simulink model "BLDC_Demo"  (R2019b)
settings: Solver=FixedStepDiscrete  StartTime=0.0  StopTime=Inf  FixedStep=0.001  RelTol=1e-3  EnableMultiTasking=on
PreLoadFcn:
  | run('BLDC_Demo_ini.m')
PostLoadFcn:
  | , if any(exist('dsrtsu_mdlpostloadfcn', 'file') ~= 0), dsrtsu_mdlpostloadfcn('Execute', bdroot); end,
InitFcn:
  | , if any(exist('rtifpga_mdlclblib', 'file') ~= 0), rtifpga_mdlclblib('Init', bdroot); end,
values from neighbouring files (symbols this model uses):
  BLDC_Ctrl_Ctrl_mode_SW = 3    [BLDC_Demo_ini.m]
  BLDC_Ctrl_iA_Set = 0    [BLDC_Demo_ini.m]
  BLDC_Ctrl_iA_Stroke = 0    [BLDC_Demo_ini.m]
  BLDC_Ctrl_is_dir = is_dir    [BLDC_Demo_ini.m]
  BLDC_Ctrl_is_index = is_index    [BLDC_Demo_ini.m]
  BLDC_Ctrl_Ki_iA = KI_i    (= 7190.04058695)    [BLDC_Demo_ini.m]
  BLDC_Ctrl_Ki_n = KI_n    (= 10.7018628664)    [BLDC_Demo_ini.m]
  BLDC_Ctrl_Kp_iA = KP_i    (= 3.09991410791)    [BLDC_Demo_ini.m]
  BLDC_Ctrl_Kp_n = KP_n    (= 0.0877769226706)    [BLDC_Demo_ini.m]
  BLDC_Ctrl_Limit_iA = IA_MAX    (= 9.5)    [BLDC_Demo_ini.m]
  BLDC_Ctrl_n_Limit = N_MAX    (= 3000)    [BLDC_Demo_ini.m]
  BLDC_Ctrl_n_Set = 0    [BLDC_Demo_ini.m]
  BLDC_Ctrl_n_Stroke = 0    [BLDC_Demo_ini.m]
  BLDC_Ctrl_TF_iA = TF_iA    (= 7.95774715459e-05)    [BLDC_Demo_ini.m]
  BLDC_Ctrl_TF_n = TF_n    (= 0.00159154943092)    [BLDC_Demo_ini.m]
  BLDC_Ctrl_v_Set = 0    [BLDC_Demo_ini.m]
  Modulator_Zi_HSD = Zi_HSD_LSD(:,4:6)    [BLDC_Demo_ini.m]
  Modulator_Zi_LSD = Zi_HSD_LSD(:,7:9)    [BLDC_Demo_ini.m]
  T_PWM = 50e-6    (= 5e-05)    [BLDC_Demo_ini.m]
undefined symbols (not defined in the file or in its folder): clock
libraries: simulink x29, rti1202lib_adc_class1 x8, dsextras x4, rtiemclib x4, rti1202lib_dio_class1 x3, rti1202lib_base x1
(part 2 of 3)

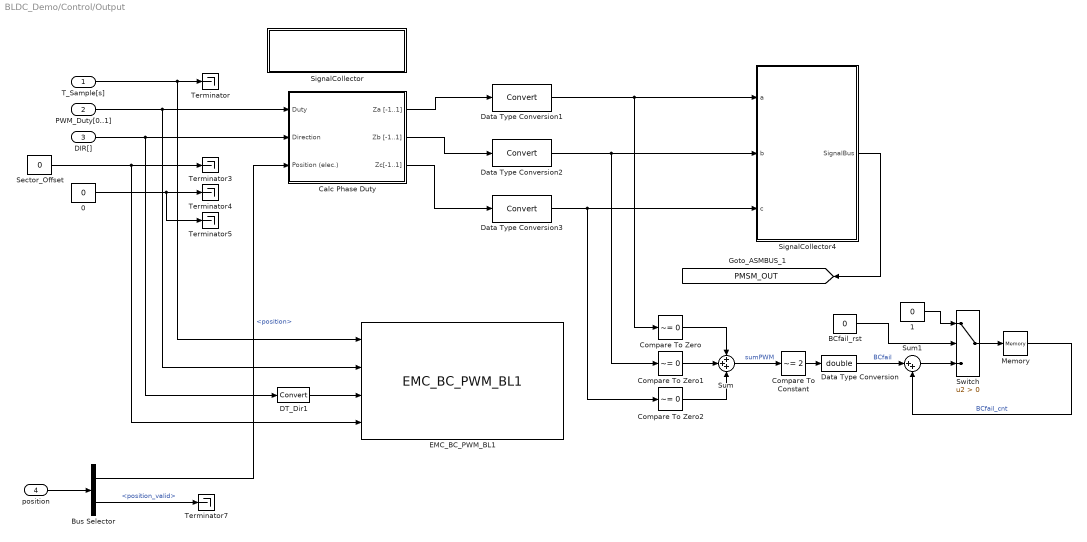
== system BLDC_Demo/Control/Output ==
  T_Sample[s] : Inport
  PWM_Duty[0..1] : Inport  Port=2
  DIR[] : Inport  Port=3
  position : Inport  Port=4
  0 : Constant  Value=0
  1 : Constant  Value=0
  BCfail_rst : Constant  Value=0
  Bus Selector : BusSelector  OutputSignals=position,position_valid
  Calc Phase Duty : Subsystem
  Compare To Constant : simulink/Logic and Bit Operations/Compare To Constant  relop=~=  const=2  OutDataTypeStr=uint8  ZeroCross=off
  Compare To Zero : simulink/Logic and Bit Operations/Compare To Zero  relop=~=  OutDataTypeStr=uint8  ZeroCross=off
  Compare To Zero1 : simulink/Logic and Bit Operations/Compare To Zero  relop=~=  OutDataTypeStr=uint8  ZeroCross=off
  Compare To Zero2 : simulink/Logic and Bit Operations/Compare To Zero  relop=~=  OutDataTypeStr=uint8  ZeroCross=off
  DT_Dir1 : DataTypeConversion
  Data Type Conversion : DataTypeConversion  OutDataTypeStr=double
  Data Type Conversion1 : DataTypeConversion
  Data Type Conversion2 : DataTypeConversion
  Data Type Conversion3 : DataTypeConversion
  EMC_BC_PWM_BL1 : rtiemclib/EMC_BC_PWM_BL1  DSProperties=struct('RTI',struct('Version',uint32(2),'BlockType',struct('isSLSource',uint8(0),'isSLSink',uint8(1),'isHWSource',uint8(0),'isHWSink',uint8(1),'isSetup',uint8(0),'isInline',uint8(1),'isNonInline',uint8(0),'isInterrupt',uint8(0),'isChannelwise',uint8(0)),'IOBoardType','DSEMC','UnitType','BCPWM','Identifier','BCPWM','DialogType','ML','BlockSet','RTIEMC','SlaveProcessor','NONE'))  RTIBlockInterface=struct('InputPortsWidth',int32([1 1 1 1 1 1 1 1]),'InputPortsActive',[1 1 1 1 0 0 0 0],'InputPortsName',{{'Period',['Duty Cycle'],'Direction','Offset','Position',['Position Valid'],['Specific Pattern'],['Output Enable']}},'InputPortsDataType',{{'SS_DOUBLE','SS_DOUBLE','SS_INT32','SS_DOUBLE','SS_DOUBLE','SS_BOOLEAN','SS_UINT32','SS_BOOLEAN'}},'BlockDisplay',{{['EMC Block Commutated PWM\nUnit: 1\nPort: 1\nChannel: 7'],'center'}},'IconTransparency','on','InitLevel',3,'DialogFcn','rtiemcbcpwmgui','BlockName',struct('Token',{{'EMC_BC_PWM_BL1'}}))  RTIBlockParameters=struct('UnitNo',{{1,'OFF',[1 2]}},'PortNo',{{1,'OFF',[1 3]}},'ChannelNo',{{7,'OFF',[1 14]}},'HighLevel',{{3,'OFF',[1 3]}},'PhaseAPos',{{[3 3 1 1 1 1],'OFF',[1 6]}},'PhaseANeg',{{[1 1 1 3 3 1],'OFF',[1 6]}},'PhaseBPos',{{[1 1 3 3 1 1],'OFF',[1 6]}},'PhaseBNeg',{{[3 1 1 1 1 3],'OFF',[1 6]}},'PhaseCPos',{{[1 1 1 1 3 3],'OFF',[1 6]}},'PhaseCNeg',{{[1 3 3 1 1 1],'OFF',[1 6]}},'UpdateMode',{{1,'OFF',[1 3]}},'DeadTime',{{'0','OFF',[0 0.000655]}},'InitPeriod',{{'5e-05','OFF',[1e-7 1.34]}},'InitDutyCycle',{{'0.5','OFF',[0 1]}},'PhaseAPosInit',{{1,'OFF',[1 2]}},'PhaseANegInit',{{1,'OFF',[1 2]}},'PhaseBPosInit',{{1,'OFF',[1 2]}},'PhaseBNegInit',{{1,'OFF',[1 2]}},'PhaseCPosInit',{{1,'OFF',[1 2]}},'PhaseCNegInit',{{1,'OFF',[1 2]}},'TerminationMode',{{0,'OFF',[0 1]}},'PhaseAPosTerm',{{1,'OFF',[1 2]}},'PhaseANegTerm',{{1,'OFF',[1 2]}},'PhaseBPosTerm',{{1,'OFF',[1 2]}},'PhaseBNegTerm',{{1,'OFF',[1 2]}},'PhaseCPosTerm',{{1,'OFF',[1 2]}},'PhaseCNegTerm',{{1,'OFF',[1 2]}},'SectorOffset',{{'0','OFF',[-60 60]}},'EnableSectorOffsetPort',{{1,'OFF',[0 1]}},'EnablePositionPort',{{1,'OFF',[1 2]}},'EnableDirectionPort',{{1,'OFF',[0 1]}},'InitDirection',{{1,'OFF',[-1 1]}},'AcuInstanceIdx',{{1,'OFF',[1 4]}},'EnableEvent',{{1,'OFF',[0 1]}},'EventMode',{{3,'OFF',[1 3]}},'EventOnStart',{{0,'OFF',[0 1]}},'EventOnCenter',{{1,'OFF',[0 1]}},'EventDelay',{{'0','OFF',[0 1.34]}},'EventRate',{{'1','OFF',[1 256]}},'TriggerLine',{{1,'OFF',[1 16]}},'TLCFileName',{{'rtiemcbcpwm','OFF',[]}},'ValidateEventBuildCheck',{{true,'OFF',[]}},'EnableSpecificPatternPort',{{0,'OFF',[0 1]}},'PhaseAPosSpecPatt',{{[1 1 1 1 1 1],'OFF',[1 6]}},'PhaseANegSpecPatt',{{[1 1 1 1 1 1],'OFF',[1 6]}},'PhaseBPosSpecPatt',{{[1 1 1 1 1 1],'OFF',[1 6]}},'PhaseBNegSpecPatt',{{[1 1 1 1 1 1],'OFF',[1 6]}},'PhaseCPosSpecPatt',{{[1 1 1 1 1 1],'OFF',[1 6]}},'PhaseCNegSpecPatt',{{[1 1 1 1 1 1],'OFF',[1 6]}},'ActivateOutputEnablePort',{{0,'OFF',[0 1]}},'InitOutputEnable',{{1,'OFF',[1 2]}})  RTISFcnParameters=struct('UnitNo','int32','PortNo','int32','ChannelNo','int32','HighLevel','int32','PhaseAPos','int32','PhaseANeg','int32','PhaseBPos','int32','PhaseBNeg','int32','PhaseCPos','int32','PhaseCNeg','int32','UpdateMode','int32','DeadTime','double','InitPeriod','double','InitDutyCycle','double','PhaseAPosInit','int32','PhaseANegInit','int32','PhaseBPosInit','int32','PhaseBNegInit','int32','PhaseCPosInit','int32','PhaseCNegInit','int32','TerminationMode','int32','PhaseAPosTerm','int32','PhaseANegTerm','int32','PhaseBPosTerm','int32','PhaseBNegTerm','int32','PhaseCPosTerm','int32','PhaseCNegTerm','int32','SectorOffset','double','EnableSectorOffsetPort','int32','EnablePositionPort','int32','EnableDirectionPort','int32','InitDirection','int32','AcuInstanceIdx','int32','EnableEvent','int32','EventMode','int32','EventOnStart','int32','EventOnCenter','int32','EventDelay','double','EventRate','int32','TriggerLine','int32','TLCFileName','char','EnableSpecificPatternPort','int32','PhaseAPosSpecPatt','int32','PhaseANegSpecPatt','int32','PhaseBPosSpecPatt','int32','PhaseBNegSpecPatt','int32','PhaseCPosSpecPatt','int32','PhaseCNegSpecPatt','int32','ActivateOutputEnablePort','int32','InitOutputEnable','int32')  RTIBlockParaDefault=struct('UnitNo',1,'PortNo',1,'ChannelNo',1,'HighLevel',1,'PhaseAPos',[3 3 1 1 1 1],'PhaseANeg',[1 1 1 3 3 1],'PhaseBPos',[1 1 3 3 1 1],'PhaseBNeg',[3 1 1 1 1 3],'PhaseCPos',[1 1 1 1 3 3],'PhaseCNeg',[1 3 3 1 1 1],'UpdateMode',1,'DeadTime',0,'InitPeriod',5e-5,'InitDutyCycle',2^-1,'PhaseAPosInit',1,'PhaseANegInit',1,'PhaseBPosInit',1,'PhaseBNegInit',1,'PhaseCPosInit',1,'PhaseCNegInit',1,'TerminationMode',0,'PhaseAPosTerm',1,'PhaseANegTerm',1,'PhaseBPosTerm',1,'PhaseBNegTerm',1,'PhaseCPosTerm',1,'PhaseCNegTerm',1,'SectorOffset',0,'EnableSectorOffsetPort',0,'EnablePositionPort',1,'EnableDirectionPort',0,'InitDirection',1,'AcuInstanceIdx',0,'EnableEvent',0,'EventMode',1,'EventOnStart',1,'EventOnCenter',0,'EventDelay',0,'EventRate',1,'TriggerLine',1,'TLCFileName','rtiemcbcpwm','ValidateEventBuildCheck',0,'EnableSpecificPatternPort',0,'PhaseAPosSpecPatt',[1 1 1 1 1 1],'PhaseANegSpecPatt',[1 1 1 1 1 1],'PhaseBPosSpecPatt',[1 1 1 1 1 1],'PhaseBNegSpecPatt',[1 1 1 1 1 1],'PhaseCPosSpecPatt',[1 1 1 1 1 1],'PhaseCNegSpecPatt',[1 1 1 1 1 1],'ActivateOutputEnablePort',0,'InitOutputEnable',1)
      settings: SourceProductName=dSPACE RTI Electric Motor Control Blockset
  Memory : Memory  InheritSampleTime=on
  Sector_Offset : Constant  Value=0
  SignalCollector : Subsystem
  SignalCollector4 : Subsystem
  Sum : Sum  Inputs=+++
  Sum1 : Sum  Inputs=|++
  Switch : Switch  Criteria=u2 > Threshold
  Terminator{,3..5,7} (5 alike) : Terminator
  tag scope: PMSM_OUT=global
  wires:
  PWM_Duty[0..1]/1 -> EMC_BC_PWM_BL1/2, Calc Phase Duty/1(Duty)
  T_Sample[s]/1 -> EMC_BC_PWM_BL1/1, Terminator/1
  SignalCollector4/1(SignalBus) -> [PMSM_OUT]
  DIR[]/1 -> DT_Dir1/1, Calc Phase Duty/2(Direction)
  Sector_Offset/1 -> Terminator3/1, EMC_BC_PWM_BL1/4
  0/1 -> Terminator5/1, Terminator4/1
  Compare To Zero1/1 -> Sum/2
  Compare To Zero/1 -> Sum/1
  Compare To Zero2/1 -> Sum/3
  Sum/1 -> Compare To Constant/1  "sumPWM"
  Compare To Constant/1 -> Data Type Conversion/1
  Memory/1 -> Sum1/2  "BCfail_cnt"
  Data Type Conversion/1 -> Sum1/1  "BCfail"
  Sum1/1 -> Switch/3
  Switch/1 -> Memory/1
  1/1 -> Switch/1
  BCfail_rst/1 -> Switch/2
  Data Type Conversion1/1 -> SignalCollector4/1(a), Compare To Zero/1
  Data Type Conversion2/1 -> SignalCollector4/2(b), Compare To Zero1/1
  Data Type Conversion3/1 -> SignalCollector4/3(c), Compare To Zero2/1
  DT_Dir1/1 -> EMC_BC_PWM_BL1/3
  position/1 -> Bus Selector/1
  Bus Selector/2 -> Terminator7/1  "<position_valid>"
  Bus Selector/1 -> Calc Phase Duty/3(Position (elec.))  "<position>"
  Calc Phase Duty/1(Za [-1..1]) -> Data Type Conversion1/1
  Calc Phase Duty/2(Zb [-1..1]) -> Data Type Conversion2/1
  Calc Phase Duty/3(Zc[-1..1]) -> Data Type Conversion3/1

== system BLDC_Demo/Control/bldc_ctrl_par_sig ==
  rect_pulse : Inport
  MDL_DISP : Subsystem
      mask Display: disp('Simulation results:\nArbitrary input to\nControlDesk from MDL')
  MDL_DISP_INPUT : Subsystem
      mask Display: disp('Simulation results:\nArbitrary input to\nControlDesk from MDL')
  MDL_OUTPUT : Subsystem
      mask Display: disp('Simulation results:\nArbitrary input to\nControlDesk from MDL')
  MDL_PAR : Subsystem
      mask Display: disp('Simulation parameters:\nContinuous output from\nControlDesk to MDL')
  wires:
  rect_pulse/1 -> MDL_PAR/1(rect_pulse)

== system BLDC_Demo/RTI Data/RTI Data Store ==
  RTI Data Store : Subsystem  mask(RTI_DATA_STORE){}
      mask help:
      | RTI Data Store Block. This block is used by RTI to store internal model dependent data. Deleting this block will result in data loss.
      |
      | NEVER DELETE, COPY, OR MODIFY THIS BLOCK!
      mask Help:
      | RTI Data Store Block. This block is used by RTI to store internal model dependent data. Deleting this block will result in data loss.
      | 
      | NEVER DELETE, COPY, OR MODIFY THIS BLOCK!
      mask Display: text(0.5, 0.5, ' ', 'HorizontalAlignment', 'center');

== system BLDC_Demo/Ref_value_gen/Enabled and Triggered Subsystem ==
  n_ref : Inport
  Constant : Constant
  Constant1 : Constant  Value=0
  Hit Crossing : HitCross  HitCrossingOffset=0.5  HitCrossingDirection=rising
  Memory : Memory  InheritSampleTime=on
  Product : Product  RndMeth=Zero
  Relational Operator : RelationalOperator  Operator=<=  OutDataTypeStr=boolean  RndMeth=Nearest
  Relational Operator1 : RelationalOperator  OutDataTypeStr=boolean  RndMeth=Nearest
  Sum : Sum  Inputs=|++
  Switch : Switch  Threshold=0.5
  Switch1 : Switch  Threshold=0.5
  load_signal_0 : Constant  Value=0
  load_signal_generator : Constant
  start_time_samples : Constant  Value=1000
  switch_out_boarder : Constant  Value=0.5
  load_ref : Outport  VectorParamsAs1DForOutWhenUnconnected=off
  wires:
  Constant/1 -> Sum/1
  Sum/1 -> Switch/3
  Constant1/1 -> Switch/1
  Switch/1 -> Relational Operator/1, Memory/1
  Hit Crossing/1 -> Switch/2
  n_ref/1 -> Hit Crossing/1, Relational Operator1/1
  start_time_samples/1 -> Relational Operator/2
  load_signal_0/1 -> Switch1/1
  Relational Operator/1 -> Switch1/2
  load_signal_generator/1 -> Switch1/3
  Switch1/1 -> Product/2
  switch_out_boarder/1 -> Relational Operator1/2
  Product/1 -> load_ref/1
  Relational Operator1/1 -> Product/1
  Memory/1 -> Sum/2

== system BLDC_Demo/Control/Control_load_machine/duty_cycle_2_torque ==
  In_duty_cycle[0..1] : Inport
  Divide : Product  Inputs=*/
  coil_resistance : Constant  Value=24
  current_2_load1 : Lookup_n-D  NumberOfTableDimensions=1  BreakpointsForDimension1=[0, 0.05, 0.1, 0.2, 0.3, 0.4]  Table=[0, 0.05, 0.2, 0.7, 1.4, 1.9]  InputSameDT=on
  duty_cycle_2_voltage : Subsystem
  Out_torque[Nm] : Outport  VectorParamsAs1DForOutWhenUnconnected=off
  wires:
  In_duty_cycle[0..1]/1 -> duty_cycle_2_voltage/1(In_duty_cycle[0..1])
  duty_cycle_2_voltage/1(Out_duty_voltage[V]) -> Divide/1
  coil_resistance/1 -> Divide/2
  current_2_load1/1 -> Out_torque[Nm]/1
  Divide/1 -> current_2_load1/1

== system BLDC_Demo/Control/Control_load_machine/torque_2_duty_cycle ==
  In_torque[Nm] : Inport
  current_2_voltage : Gain  Gain=24
  load_2_current4 : Lookup_n-D  NumberOfTableDimensions=1  BreakpointsForDimension1=[0, 0.05, 0.2, 0.7, 1.4, 1.9]  Table=[0, 0.05, 0.1, 0.2, 0.3, 0.4]  InputSameDT=on
  voltage_2_duty_cycle : Subsystem
  Out_duty_cycle[0..1] : Outport  VectorParamsAs1DForOutWhenUnconnected=off
  wires:
  load_2_current4/1 -> current_2_voltage/1
  current_2_voltage/1 -> voltage_2_duty_cycle/1(In_voltage[V])
  In_torque[Nm]/1 -> load_2_current4/1
  voltage_2_duty_cycle/1(Out_duty_cycle) -> Out_duty_cycle[0..1]/1

== system BLDC_Demo/Control/Control_load_machine/torque_2_duty_cycle1 ==
  In_torque[Nm] : Inport
  current_2_voltage : Gain  Gain=24
  load_2_current4 : Lookup_n-D  NumberOfTableDimensions=1  BreakpointsForDimension1=[0, 0.05, 0.2, 0.7, 1.4, 1.9]  Table=[0, 0.05, 0.1, 0.2, 0.3, 0.4]  InputSameDT=on
  voltage_2_duty_cycle : Subsystem
  Out_duty_cycle[0..1] : Outport  VectorParamsAs1DForOutWhenUnconnected=off
  wires:
  voltage_2_duty_cycle/1(Out_duty_cycle[0..1]) -> Out_duty_cycle[0..1]/1
  In_torque[Nm]/1 -> load_2_current4/1
  current_2_voltage/1 -> voltage_2_duty_cycle/1(In_voltage[V])
  load_2_current4/1 -> current_2_voltage/1

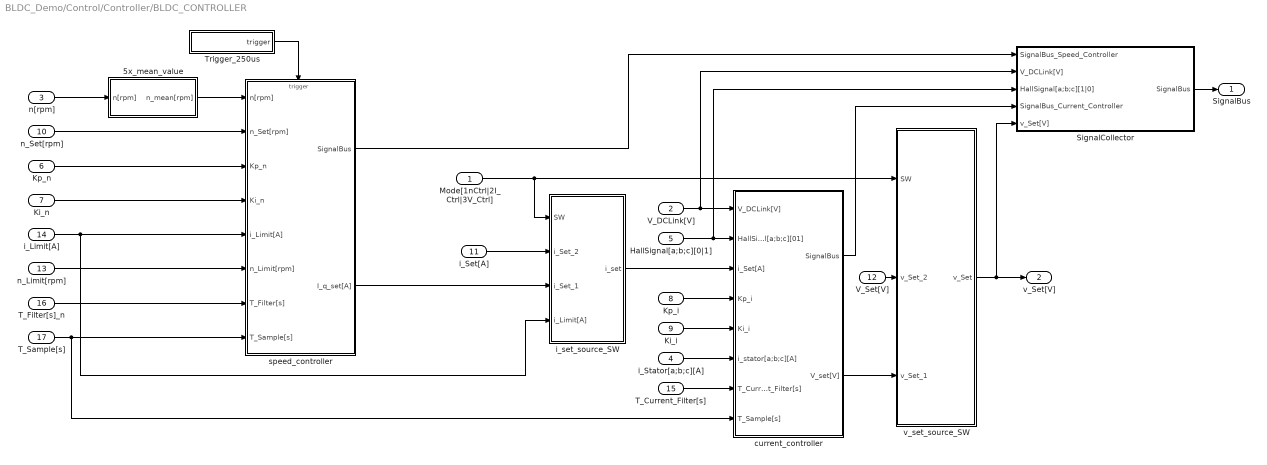
== system BLDC_Demo/Control/Controller/BLDC_CONTROLLER ==
  Mode[1nCtrl|2I_Ctrl|3V_Ctrl] : Inport
  V_DCLink[V] : Inport  Port=2
  n[rpm] : Inport  Port=3
  i_Stator[a;b;c][A] : Inport  Port=4
  HallSignal[a;b;c][0|1] : Inport  Port=5
  Kp_n : Inport  Port=6
  Ki_n : Inport  Port=7
  Kp_i : Inport  Port=8
  Ki_i : Inport  Port=9
  n_Set[rpm] : Inport  Port=10
  i_Set[A] : Inport  Port=11
  V_Set[V] : Inport  Port=12
  n_Limit[rpm] : Inport  Port=13
  i_Limit[A] : Inport  Port=14
  T_Current_Filter[s] : Inport  Port=15
  T_Filter[s]_n : Inport  Port=16
  T_Sample[s] : Inport  Port=17
  5x_mean_value : Subsystem
  SignalCollector : Subsystem
  Trigger_250us : Subsystem
  current_controller : Subsystem
  i_set_source_SW : Subsystem
  speed_controller : Subsystem
  v_set_source_SW : Subsystem
  SignalBus : Outport  VectorParamsAs1DForOutWhenUnconnected=off
  v_Set[V] : Outport  Port=2  VectorParamsAs1DForOutWhenUnconnected=off
  wires:
  T_Sample[s]/1 -> current_controller/8(T_Sample[s]), speed_controller/8(T_Sample[s])
  i_Limit[A]/1 -> i_set_source_SW/4(i_Limit[A]), speed_controller/5(i_Limit[A])
  Ki_n/1 -> speed_controller/4(Ki_n)
  Kp_n/1 -> speed_controller/3(Kp_n)
  n[rpm]/1 -> 5x_mean_value/1(n[rpm])
  n_Set[rpm]/1 -> speed_controller/2(n_Set[rpm])
  n_Limit[rpm]/1 -> speed_controller/6(n_Limit[rpm])
  V_DCLink[V]/1 -> SignalCollector/2(V_DCLink[V]), current_controller/1(V_DCLink[V])
  T_Current_Filter[s]/1 -> current_controller/7(T_Current_Filter[s])
  HallSignal[a;b;c][0|1]/1 -> SignalCollector/3(HallSignal[a;b;c][1|0]), current_controller/2(HallSignal[a;b;c][01])
  i_Stator[a;b;c][A]/1 -> current_controller/6(i_stator[a;b;c][A])
  v_set_source_SW/1(v_Set) -> v_Set[V]/1, SignalCollector/5(v_Set[V])
  current_controller/2(" V_set[V]") -> v_set_source_SW/3(v_Set_1)
  V_Set[V]/1 -> v_set_source_SW/2(v_Set_2)
  speed_controller/2(I_q_set[A]) -> i_set_source_SW/3(i_Set_1)
  i_Set[A]/1 -> i_set_source_SW/2(i_Set_2)
  Ki_i/1 -> current_controller/5(Ki_i)
  Kp_i/1 -> current_controller/4(Kp_i)
  SignalCollector/1(SignalBus) -> SignalBus/1
  i_set_source_SW/1(i_set) -> current_controller/3(i_Set[A])
  Mode[1nCtrl|2I_Ctrl|3V_Ctrl]/1 -> i_set_source_SW/1(SW), v_set_source_SW/1(SW)
  current_controller/1(SignalBus) -> SignalCollector/4(SignalBus_Current_Controller)
  speed_controller/1(SignalBus) -> SignalCollector/1(SignalBus_Speed_Controller)
  T_Filter[s]_n/1 -> speed_controller/7(T_Filter[s])
  5x_mean_value/1(n_mean[rpm]) -> speed_controller/1(n[rpm])
  Trigger_250us/1(trigger) -> speed_controller/Trigger

== system BLDC_Demo/Control/Controller/BLOCK_MODULATOR ==
  V_DCLink[V] : Inport
  v_Set[V] : Inport  Port=2
  HallSignal[a;b;c][0|1] : Inport  Port=3
  Data Type Conversion : DataTypeConversion  OutDataTypeStr=double
  Data Type Conversion1 : DataTypeConversion  OutDataTypeStr=double
  DutyCycle : Subsystem
  Label_DutyCycle_HSD[a;b;c][0_1] : Subsystem
  Label_DutyCycle_LSD[a;b;c][0_1] : Subsystem
  Product1 : Product  RndMeth=Zero
  SignalCollector : Subsystem
  SwitchHSD : Switch
  SwitchLSD : Switch
  Zabc_HSD : CombinatorialLogic  TruthTable=Zi_HSD
  Zabc_LSD : CombinatorialLogic  TruthTable=Zi_LSD
  SignalBus : Outport  VectorParamsAs1DForOutWhenUnconnected=off
  d[0_1] : Outport  Port=2  VectorParamsAs1DForOutWhenUnconnected=off
  DIR : Outport  Port=3  VectorParamsAs1DForOutWhenUnconnected=off
  wires:
  v_Set[V]/1 -> DutyCycle/1(v_set[V])
  V_DCLink[V]/1 -> DutyCycle/2(V_DCLink[V])
  DutyCycle/2(DIR) -> SwitchHSD/2, SwitchLSD/2, SignalCollector/2(DIR), DIR/1
  DutyCycle/1(d[0_1]) -> Product1/1, SignalCollector/1(d[0_1]), d[0_1]/1
  SignalCollector/1(SignalBus) -> SignalBus/1
  HallSignal[a;b;c][0|1]/1 -> Zabc_HSD/1, Zabc_LSD/1
  Zabc_LSD/1 -> Data Type Conversion/1
  Zabc_HSD/1 -> Data Type Conversion1/1
  SwitchHSD/1 -> Product1/2
  Data Type Conversion/1 -> SwitchLSD/1, SwitchHSD/3
  Data Type Conversion1/1 -> SwitchHSD/1, SwitchLSD/3
  Label_DutyCycle_HSD[a;b;c][0_1]/1(Out) -> SignalCollector/3(DutyCycle_HSD[a;b;c][0_1])
  Label_DutyCycle_LSD[a;b;c][0_1]/1(Out) -> SignalCollector/4(DutyCycle_LSD[a;b;c][0_1])
  Product1/1 -> Label_DutyCycle_HSD[a;b;c][0_1]/1(In)
  SwitchLSD/1 -> Label_DutyCycle_LSD[a;b;c][0_1]/1(In)

== system BLDC_Demo/Control/Controller/SignalCollector ==
  BusCreator : BusCreator  Inputs=1
  tag scope: Controller_Bus=global
  wires:
  [PMSM_CONTROLLER] -> BusCreator/1
  BusCreator/1 -> [Controller_Bus]  "Controller"

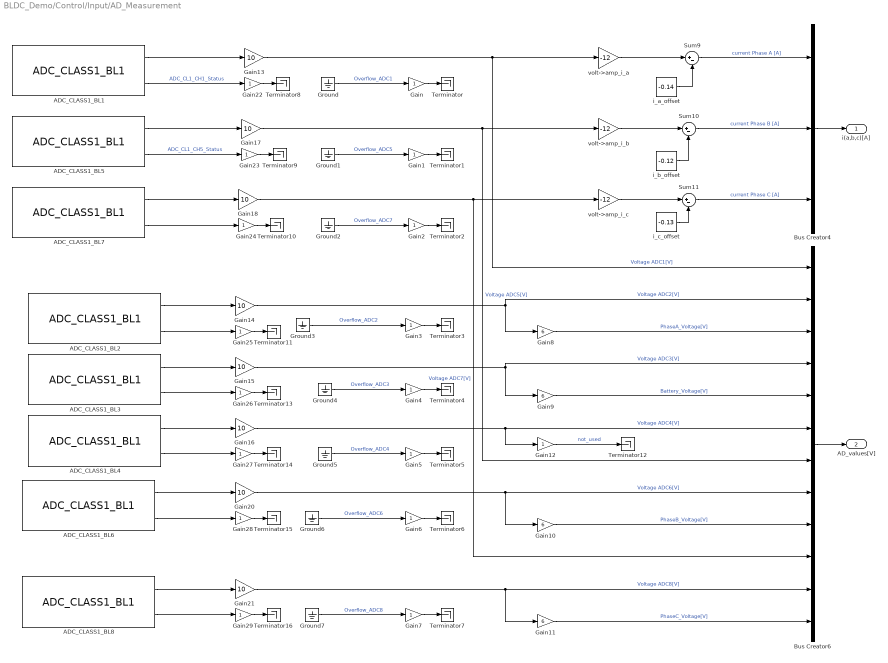
== system BLDC_Demo/Control/Input/AD_Measurement ==
  " i_a_offset" : Constant  Value=-0.14
  " i_b_offset  " : Constant  Value=-0.12
  ADC_CLASS1_BL1 : rti1202lib_adc_class1/ADC_CLASS1_BL1  DSProperties=struct('RTI',struct('Version',uint32(1),'BlockType',struct('isSLSource',uint8(1),'isSLSink',uint8(1),'isHWSource',uint8(0),'isHWSink',uint8(1),'isSetup',uint8(0),'isInline',uint8(1),'isNonInline',uint8(0),'isInterrupt',uint8(0),'isChannelwise',uint8(1)),'IOBoardType',{{'DS120X','STD','ADCC1'}},'UnitType','ADC','Identifier','ADC','DialogType','ML','BlockSet','NONE','SlaveProcessor','NONE'))  RTIBlockInterface=struct('InputPortsActive',0,'InputPortsWidth',int32(1),'InputPortsDataType',{{'SS_BOOLEAN'}},'InputPortsName',{{'Continue'}},'OutputPortsActive',[1 1],'OutputPortsWidth',int32([1 1]),'OutputPortsDataType',{{'SS_DOUBLE','SS_INT16'}},'OutputPortsName',{{'ADC','Status'}},'DialogFcn','rti120xstdadcc1adcgui','SampleTime',{{-1}},'InitLevel',3,'IconTransparency','on','BlockDisplay',{{['ADC CL1\nChannel: 1'],'center'}},'BlockName',struct('Token',{{'ADC_CLASS1_BL1'}}))  RTIBlockParameters=struct('ReadMode',{{2,'OFF',[1 2]}},'ChannelNo',{{1,'OFF',[]}},'ConversionMode',{{1,'OFF',[1 2]}},'TriggerSource',{{2,'OFF',[1 2]}},'TriggerLineIn',{{1,'OFF',[1 16]}},'SampleMode',{{1,'OFF',[1 2]}},'BurstTriggerSource',{{1,'OFF',[1 2]}},'BurstTriggerLine',{{1,'OFF',[1 16]}},'ConvTriggerSource',{{3,'OFF',[1 3]}},'ConvTriggerLine',{{1,'OFF',[1 16]}},'ConvPeriod',{{'100e-6','OFF',[1e-6 1.34]}},'ConvPeriodCheck',{{0,'OFF',[]}},'BurstSize',{{'10','OFF',[]}},'BurstSizeCheck',{{0,'OFF',[]}},'DataSetOffset',{{'0','OFF',[]}},'DataSetOffsetCheck',{{0,'OFF',[]}},'DataSetLength',{{'1','OFF',[]}},'DataSetLengthCheck',{{0,'OFF',[]}},'EnableTriggerEvent',{{0,'OFF',[0 1]}},'TriggerMode',{{2,'OFF',[1 3]}},'TriggerLineOut',{{1,'OFF',[1 16]}},'ADCSWStartEnable',{{0,'OFF',[0 1]}},'SampleTime',{{'-1','OFF',[-1 inf]}},'SampleTimeCheck',{{0,'OFF',[]}},'StatusPortEnable',{{1,'OFF',[0 1]}},'TLCFileName',{{'rti120xadc_c1_adc','OFF',[]}})  RTISFcnParameters=struct('ReadMode','int16','ChannelNo','int16','ConversionMode','int16','TriggerSource','int16','TriggerLineIn','int16','SampleMode','int16','BurstTriggerSource','int16','BurstTriggerLine','int16','ConvTriggerSource','int16','ConvTriggerLine','int16','ConvPeriod','double','BurstSize','int16','DataSetOffset','int16','DataSetLength','int16','EnableTriggerEvent','int16','TriggerMode','int16','TriggerLineOut','int16','ADCSWStartEnable','int16','SampleTime','double','StatusPortEnable','int16','TLCFileName','char')  RTIBlockParaDefault=struct('ReadMode',1,'ChannelNo',1,'ConversionMode',1,'TriggerSource',1,'TriggerLineIn',1,'SampleMode',1,'BurstTriggerSource',1,'BurstTriggerLine',1,'ConvTriggerSource',3,'ConvTriggerLine',1,'ConvPeriod',0.0001,'ConvPeriodCheck',0,'BurstSize',10,'BurstSizeCheck',0,'DataSetOffset',0,'DataSetOffsetCheck',0,'DataSetLength',1,'DataSetLengthCheck',0,'EnableTriggerEvent',0,'TriggerMode',2,'TriggerLineOut',1,'ADCSWStartEnable',0,'SampleTime',-1,'SampleTimeCheck',1,'StatusPortEnable',0,'TLCFileName','rti120xadc_c1_adc')
  ADC_CLASS1_BL2 : rti1202lib_adc_class1/ADC_CLASS1_BL1  DSProperties=struct('RTI',struct('Version',uint32(1),'BlockType',struct('isSLSource',uint8(1),'isSLSink',uint8(1),'isHWSource',uint8(0),'isHWSink',uint8(1),'isSetup',uint8(0),'isInline',uint8(1),'isNonInline',uint8(0),'isInterrupt',uint8(0),'isChannelwise',uint8(1)),'IOBoardType',{{'DS120X','STD','ADCC1'}},'UnitType','ADC','Identifier','ADC','DialogType','ML','BlockSet','NONE','SlaveProcessor','NONE'))  RTIBlockInterface=struct('InputPortsActive',0,'InputPortsWidth',int32(1),'InputPortsDataType',{{'SS_BOOLEAN'}},'InputPortsName',{{'Continue'}},'OutputPortsActive',[1 1],'OutputPortsWidth',int32([1 1]),'OutputPortsDataType',{{'SS_DOUBLE','SS_INT16'}},'OutputPortsName',{{'ADC','Status'}},'DialogFcn','rti120xstdadcc1adcgui','SampleTime',{{-1}},'InitLevel',3,'IconTransparency','on','BlockDisplay',{{['ADC CL1\nChannel: 2'],'center'}},'BlockName',struct('Token',{{'ADC_CLASS1_BL1'}}))  RTIBlockParameters=struct('ReadMode',{{2,'OFF',[1 2]}},'ChannelNo',{{2,'OFF',[]}},'ConversionMode',{{1,'OFF',[1 2]}},'TriggerSource',{{2,'OFF',[1 2]}},'TriggerLineIn',{{1,'OFF',[1 16]}},'SampleMode',{{1,'OFF',[1 2]}},'BurstTriggerSource',{{1,'OFF',[1 2]}},'BurstTriggerLine',{{1,'OFF',[1 16]}},'ConvTriggerSource',{{3,'OFF',[1 3]}},'ConvTriggerLine',{{1,'OFF',[1 16]}},'ConvPeriod',{{'100e-6','OFF',[1e-6 1.34]}},'ConvPeriodCheck',{{0,'OFF',[]}},'BurstSize',{{'10','OFF',[]}},'BurstSizeCheck',{{0,'OFF',[]}},'DataSetOffset',{{'0','OFF',[]}},'DataSetOffsetCheck',{{0,'OFF',[]}},'DataSetLength',{{'1','OFF',[]}},'DataSetLengthCheck',{{0,'OFF',[]}},'EnableTriggerEvent',{{0,'OFF',[0 1]}},'TriggerMode',{{2,'OFF',[1 3]}},'TriggerLineOut',{{1,'OFF',[1 16]}},'ADCSWStartEnable',{{0,'OFF',[0 1]}},'SampleTime',{{'-1','OFF',[-1 inf]}},'SampleTimeCheck',{{0,'OFF',[]}},'StatusPortEnable',{{1,'OFF',[0 1]}},'TLCFileName',{{'rti120xadc_c1_adc','OFF',[]}})  RTISFcnParameters=struct('ReadMode','int16','ChannelNo','int16','ConversionMode','int16','TriggerSource','int16','TriggerLineIn','int16','SampleMode','int16','BurstTriggerSource','int16','BurstTriggerLine','int16','ConvTriggerSource','int16','ConvTriggerLine','int16','ConvPeriod','double','BurstSize','int16','DataSetOffset','int16','DataSetLength','int16','EnableTriggerEvent','int16','TriggerMode','int16','TriggerLineOut','int16','ADCSWStartEnable','int16','SampleTime','double','StatusPortEnable','int16','TLCFileName','char')  RTIBlockParaDefault=struct('ReadMode',1,'ChannelNo',1,'ConversionMode',1,'TriggerSource',1,'TriggerLineIn',1,'SampleMode',1,'BurstTriggerSource',1,'BurstTriggerLine',1,'ConvTriggerSource',3,'ConvTriggerLine',1,'ConvPeriod',0.0001,'ConvPeriodCheck',0,'BurstSize',10,'BurstSizeCheck',0,'DataSetOffset',0,'DataSetOffsetCheck',0,'DataSetLength',1,'DataSetLengthCheck',0,'EnableTriggerEvent',0,'TriggerMode',2,'TriggerLineOut',1,'ADCSWStartEnable',0,'SampleTime',-1,'SampleTimeCheck',1,'StatusPortEnable',0,'TLCFileName','rti120xadc_c1_adc')
  ADC_CLASS1_BL3 : rti1202lib_adc_class1/ADC_CLASS1_BL1  DSProperties=struct('RTI',struct('Version',uint32(1),'BlockType',struct('isSLSource',uint8(1),'isSLSink',uint8(1),'isHWSource',uint8(0),'isHWSink',uint8(1),'isSetup',uint8(0),'isInline',uint8(1),'isNonInline',uint8(0),'isInterrupt',uint8(0),'isChannelwise',uint8(1)),'IOBoardType',{{'DS120X','STD','ADCC1'}},'UnitType','ADC','Identifier','ADC','DialogType','ML','BlockSet','NONE','SlaveProcessor','NONE'))  RTIBlockInterface=struct('InputPortsActive',0,'InputPortsWidth',int32(1),'InputPortsDataType',{{'SS_BOOLEAN'}},'InputPortsName',{{'Continue'}},'OutputPortsActive',[1 1],'OutputPortsWidth',int32([1 1]),'OutputPortsDataType',{{'SS_DOUBLE','SS_INT16'}},'OutputPortsName',{{'ADC','Status'}},'DialogFcn','rti120xstdadcc1adcgui','SampleTime',{{-1}},'InitLevel',3,'IconTransparency','on','BlockDisplay',{{['ADC CL1\nChannel: 3'],'center'}},'BlockName',struct('Token',{{'ADC_CLASS1_BL1'}}))  RTIBlockParameters=struct('ReadMode',{{2,'OFF',[1 2]}},'ChannelNo',{{3,'OFF',[]}},'ConversionMode',{{1,'OFF',[1 2]}},'TriggerSource',{{2,'OFF',[1 2]}},'TriggerLineIn',{{1,'OFF',[1 16]}},'SampleMode',{{1,'OFF',[1 2]}},'BurstTriggerSource',{{1,'OFF',[1 2]}},'BurstTriggerLine',{{1,'OFF',[1 16]}},'ConvTriggerSource',{{3,'OFF',[1 3]}},'ConvTriggerLine',{{1,'OFF',[1 16]}},'ConvPeriod',{{'100e-6','OFF',[1e-6 1.34]}},'ConvPeriodCheck',{{0,'OFF',[]}},'BurstSize',{{'10','OFF',[]}},'BurstSizeCheck',{{0,'OFF',[]}},'DataSetOffset',{{'0','OFF',[]}},'DataSetOffsetCheck',{{0,'OFF',[]}},'DataSetLength',{{'1','OFF',[]}},'DataSetLengthCheck',{{0,'OFF',[]}},'EnableTriggerEvent',{{0,'OFF',[0 1]}},'TriggerMode',{{2,'OFF',[1 3]}},'TriggerLineOut',{{1,'OFF',[1 16]}},'ADCSWStartEnable',{{0,'OFF',[0 1]}},'SampleTime',{{'-1','OFF',[-1 inf]}},'SampleTimeCheck',{{0,'OFF',[]}},'StatusPortEnable',{{1,'OFF',[0 1]}},'TLCFileName',{{'rti120xadc_c1_adc','OFF',[]}})  RTISFcnParameters=struct('ReadMode','int16','ChannelNo','int16','ConversionMode','int16','TriggerSource','int16','TriggerLineIn','int16','SampleMode','int16','BurstTriggerSource','int16','BurstTriggerLine','int16','ConvTriggerSource','int16','ConvTriggerLine','int16','ConvPeriod','double','BurstSize','int16','DataSetOffset','int16','DataSetLength','int16','EnableTriggerEvent','int16','TriggerMode','int16','TriggerLineOut','int16','ADCSWStartEnable','int16','SampleTime','double','StatusPortEnable','int16','TLCFileName','char')  RTIBlockParaDefault=struct('ReadMode',1,'ChannelNo',1,'ConversionMode',1,'TriggerSource',1,'TriggerLineIn',1,'SampleMode',1,'BurstTriggerSource',1,'BurstTriggerLine',1,'ConvTriggerSource',3,'ConvTriggerLine',1,'ConvPeriod',0.0001,'ConvPeriodCheck',0,'BurstSize',10,'BurstSizeCheck',0,'DataSetOffset',0,'DataSetOffsetCheck',0,'DataSetLength',1,'DataSetLengthCheck',0,'EnableTriggerEvent',0,'TriggerMode',2,'TriggerLineOut',1,'ADCSWStartEnable',0,'SampleTime',-1,'SampleTimeCheck',1,'StatusPortEnable',0,'TLCFileName','rti120xadc_c1_adc')
  ADC_CLASS1_BL4 : rti1202lib_adc_class1/ADC_CLASS1_BL1  DSProperties=struct('RTI',struct('Version',uint32(1),'BlockType',struct('isSLSource',uint8(1),'isSLSink',uint8(1),'isHWSource',uint8(0),'isHWSink',uint8(1),'isSetup',uint8(0),'isInline',uint8(1),'isNonInline',uint8(0),'isInterrupt',uint8(0),'isChannelwise',uint8(1)),'IOBoardType',{{'DS120X','STD','ADCC1'}},'UnitType','ADC','Identifier','ADC','DialogType','ML','BlockSet','NONE','SlaveProcessor','NONE'))  RTIBlockInterface=struct('InputPortsActive',0,'InputPortsWidth',int32(1),'InputPortsDataType',{{'SS_BOOLEAN'}},'InputPortsName',{{'Continue'}},'OutputPortsActive',[1 1],'OutputPortsWidth',int32([1 1]),'OutputPortsDataType',{{'SS_DOUBLE','SS_INT16'}},'OutputPortsName',{{'ADC','Status'}},'DialogFcn','rti120xstdadcc1adcgui','SampleTime',{{-1}},'InitLevel',3,'IconTransparency','on','BlockDisplay',{{['ADC CL1\nChannel: 4'],'center'}},'BlockName',struct('Token',{{'ADC_CLASS1_BL1'}}))  RTIBlockParameters=struct('ReadMode',{{2,'OFF',[1 2]}},'ChannelNo',{{4,'OFF',[]}},'ConversionMode',{{1,'OFF',[1 2]}},'TriggerSource',{{2,'OFF',[1 2]}},'TriggerLineIn',{{1,'OFF',[1 16]}},'SampleMode',{{1,'OFF',[1 2]}},'BurstTriggerSource',{{1,'OFF',[1 2]}},'BurstTriggerLine',{{1,'OFF',[1 16]}},'ConvTriggerSource',{{3,'OFF',[1 3]}},'ConvTriggerLine',{{1,'OFF',[1 16]}},'ConvPeriod',{{'100e-6','OFF',[1e-6 1.34]}},'ConvPeriodCheck',{{0,'OFF',[]}},'BurstSize',{{'10','OFF',[]}},'BurstSizeCheck',{{0,'OFF',[]}},'DataSetOffset',{{'0','OFF',[]}},'DataSetOffsetCheck',{{0,'OFF',[]}},'DataSetLength',{{'1','OFF',[]}},'DataSetLengthCheck',{{0,'OFF',[]}},'EnableTriggerEvent',{{0,'OFF',[0 1]}},'TriggerMode',{{2,'OFF',[1 3]}},'TriggerLineOut',{{1,'OFF',[1 16]}},'ADCSWStartEnable',{{0,'OFF',[0 1]}},'SampleTime',{{'-1','OFF',[-1 inf]}},'SampleTimeCheck',{{0,'OFF',[]}},'StatusPortEnable',{{1,'OFF',[0 1]}},'TLCFileName',{{'rti120xadc_c1_adc','OFF',[]}})  RTISFcnParameters=struct('ReadMode','int16','ChannelNo','int16','ConversionMode','int16','TriggerSource','int16','TriggerLineIn','int16','SampleMode','int16','BurstTriggerSource','int16','BurstTriggerLine','int16','ConvTriggerSource','int16','ConvTriggerLine','int16','ConvPeriod','double','BurstSize','int16','DataSetOffset','int16','DataSetLength','int16','EnableTriggerEvent','int16','TriggerMode','int16','TriggerLineOut','int16','ADCSWStartEnable','int16','SampleTime','double','StatusPortEnable','int16','TLCFileName','char')  RTIBlockParaDefault=struct('ReadMode',1,'ChannelNo',1,'ConversionMode',1,'TriggerSource',1,'TriggerLineIn',1,'SampleMode',1,'BurstTriggerSource',1,'BurstTriggerLine',1,'ConvTriggerSource',3,'ConvTriggerLine',1,'ConvPeriod',0.0001,'ConvPeriodCheck',0,'BurstSize',10,'BurstSizeCheck',0,'DataSetOffset',0,'DataSetOffsetCheck',0,'DataSetLength',1,'DataSetLengthCheck',0,'EnableTriggerEvent',0,'TriggerMode',2,'TriggerLineOut',1,'ADCSWStartEnable',0,'SampleTime',-1,'SampleTimeCheck',1,'StatusPortEnable',0,'TLCFileName','rti120xadc_c1_adc')
  ADC_CLASS1_BL5 : rti1202lib_adc_class1/ADC_CLASS1_BL1  DSProperties=struct('RTI',struct('Version',uint32(1),'BlockType',struct('isSLSource',uint8(1),'isSLSink',uint8(1),'isHWSource',uint8(0),'isHWSink',uint8(1),'isSetup',uint8(0),'isInline',uint8(1),'isNonInline',uint8(0),'isInterrupt',uint8(0),'isChannelwise',uint8(1)),'IOBoardType',{{'DS120X','STD','ADCC1'}},'UnitType','ADC','Identifier','ADC','DialogType','ML','BlockSet','NONE','SlaveProcessor','NONE'))  RTIBlockInterface=struct('InputPortsActive',0,'InputPortsWidth',int32(1),'InputPortsDataType',{{'SS_BOOLEAN'}},'InputPortsName',{{'Continue'}},'OutputPortsActive',[1 1],'OutputPortsWidth',int32([1 1]),'OutputPortsDataType',{{'SS_DOUBLE','SS_INT16'}},'OutputPortsName',{{'ADC','Status'}},'DialogFcn','rti120xstdadcc1adcgui','SampleTime',{{-1}},'InitLevel',3,'IconTransparency','on','BlockDisplay',{{['ADC CL1\nChannel: 5'],'center'}},'BlockName',struct('Token',{{'ADC_CLASS1_BL1'}}))  RTIBlockParameters=struct('ReadMode',{{2,'OFF',[1 2]}},'ChannelNo',{{5,'OFF',[]}},'ConversionMode',{{1,'OFF',[1 2]}},'TriggerSource',{{2,'OFF',[1 2]}},'TriggerLineIn',{{1,'OFF',[1 16]}},'SampleMode',{{1,'OFF',[1 2]}},'BurstTriggerSource',{{1,'OFF',[1 2]}},'BurstTriggerLine',{{1,'OFF',[1 16]}},'ConvTriggerSource',{{3,'OFF',[1 3]}},'ConvTriggerLine',{{1,'OFF',[1 16]}},'ConvPeriod',{{'100e-6','OFF',[1e-6 1.34]}},'ConvPeriodCheck',{{0,'OFF',[]}},'BurstSize',{{'10','OFF',[]}},'BurstSizeCheck',{{0,'OFF',[]}},'DataSetOffset',{{'0','OFF',[]}},'DataSetOffsetCheck',{{0,'OFF',[]}},'DataSetLength',{{'1','OFF',[]}},'DataSetLengthCheck',{{0,'OFF',[]}},'EnableTriggerEvent',{{0,'OFF',[0 1]}},'TriggerMode',{{2,'OFF',[1 3]}},'TriggerLineOut',{{1,'OFF',[1 16]}},'ADCSWStartEnable',{{0,'OFF',[0 1]}},'SampleTime',{{'-1','OFF',[-1 inf]}},'SampleTimeCheck',{{0,'OFF',[]}},'StatusPortEnable',{{1,'OFF',[0 1]}},'TLCFileName',{{'rti120xadc_c1_adc','OFF',[]}})  RTISFcnParameters=struct('ReadMode','int16','ChannelNo','int16','ConversionMode','int16','TriggerSource','int16','TriggerLineIn','int16','SampleMode','int16','BurstTriggerSource','int16','BurstTriggerLine','int16','ConvTriggerSource','int16','ConvTriggerLine','int16','ConvPeriod','double','BurstSize','int16','DataSetOffset','int16','DataSetLength','int16','EnableTriggerEvent','int16','TriggerMode','int16','TriggerLineOut','int16','ADCSWStartEnable','int16','SampleTime','double','StatusPortEnable','int16','TLCFileName','char')  RTIBlockParaDefault=struct('ReadMode',1,'ChannelNo',1,'ConversionMode',1,'TriggerSource',1,'TriggerLineIn',1,'SampleMode',1,'BurstTriggerSource',1,'BurstTriggerLine',1,'ConvTriggerSource',3,'ConvTriggerLine',1,'ConvPeriod',0.0001,'ConvPeriodCheck',0,'BurstSize',10,'BurstSizeCheck',0,'DataSetOffset',0,'DataSetOffsetCheck',0,'DataSetLength',1,'DataSetLengthCheck',0,'EnableTriggerEvent',0,'TriggerMode',2,'TriggerLineOut',1,'ADCSWStartEnable',0,'SampleTime',-1,'SampleTimeCheck',1,'StatusPortEnable',0,'TLCFileName','rti120xadc_c1_adc')
  ADC_CLASS1_BL6 : rti1202lib_adc_class1/ADC_CLASS1_BL1  DSProperties=struct('RTI',struct('Version',uint32(1),'BlockType',struct('isSLSource',uint8(1),'isSLSink',uint8(1),'isHWSource',uint8(0),'isHWSink',uint8(1),'isSetup',uint8(0),'isInline',uint8(1),'isNonInline',uint8(0),'isInterrupt',uint8(0),'isChannelwise',uint8(1)),'IOBoardType',{{'DS120X','STD','ADCC1'}},'UnitType','ADC','Identifier','ADC','DialogType','ML','BlockSet','NONE','SlaveProcessor','NONE'))  RTIBlockInterface=struct('InputPortsActive',0,'InputPortsWidth',int32(1),'InputPortsDataType',{{'SS_BOOLEAN'}},'InputPortsName',{{'Continue'}},'OutputPortsActive',[1 1],'OutputPortsWidth',int32([1 1]),'OutputPortsDataType',{{'SS_DOUBLE','SS_INT16'}},'OutputPortsName',{{'ADC','Status'}},'DialogFcn','rti120xstdadcc1adcgui','SampleTime',{{-1}},'InitLevel',3,'IconTransparency','on','BlockDisplay',{{['ADC CL1\nChannel: 6'],'center'}},'BlockName',struct('Token',{{'ADC_CLASS1_BL1'}}))  RTIBlockParameters=struct('ReadMode',{{2,'OFF',[1 2]}},'ChannelNo',{{6,'OFF',[]}},'ConversionMode',{{1,'OFF',[1 2]}},'TriggerSource',{{2,'OFF',[1 2]}},'TriggerLineIn',{{1,'OFF',[1 16]}},'SampleMode',{{1,'OFF',[1 2]}},'BurstTriggerSource',{{1,'OFF',[1 2]}},'BurstTriggerLine',{{1,'OFF',[1 16]}},'ConvTriggerSource',{{3,'OFF',[1 3]}},'ConvTriggerLine',{{1,'OFF',[1 16]}},'ConvPeriod',{{'100e-6','OFF',[1e-6 1.34]}},'ConvPeriodCheck',{{0,'OFF',[]}},'BurstSize',{{'10','OFF',[]}},'BurstSizeCheck',{{0,'OFF',[]}},'DataSetOffset',{{'0','OFF',[]}},'DataSetOffsetCheck',{{0,'OFF',[]}},'DataSetLength',{{'1','OFF',[]}},'DataSetLengthCheck',{{0,'OFF',[]}},'EnableTriggerEvent',{{0,'OFF',[0 1]}},'TriggerMode',{{2,'OFF',[1 3]}},'TriggerLineOut',{{1,'OFF',[1 16]}},'ADCSWStartEnable',{{0,'OFF',[0 1]}},'SampleTime',{{'-1','OFF',[-1 inf]}},'SampleTimeCheck',{{0,'OFF',[]}},'StatusPortEnable',{{1,'OFF',[0 1]}},'TLCFileName',{{'rti120xadc_c1_adc','OFF',[]}})  RTISFcnParameters=struct('ReadMode','int16','ChannelNo','int16','ConversionMode','int16','TriggerSource','int16','TriggerLineIn','int16','SampleMode','int16','BurstTriggerSource','int16','BurstTriggerLine','int16','ConvTriggerSource','int16','ConvTriggerLine','int16','ConvPeriod','double','BurstSize','int16','DataSetOffset','int16','DataSetLength','int16','EnableTriggerEvent','int16','TriggerMode','int16','TriggerLineOut','int16','ADCSWStartEnable','int16','SampleTime','double','StatusPortEnable','int16','TLCFileName','char')  RTIBlockParaDefault=struct('ReadMode',1,'ChannelNo',1,'ConversionMode',1,'TriggerSource',1,'TriggerLineIn',1,'SampleMode',1,'BurstTriggerSource',1,'BurstTriggerLine',1,'ConvTriggerSource',3,'ConvTriggerLine',1,'ConvPeriod',0.0001,'ConvPeriodCheck',0,'BurstSize',10,'BurstSizeCheck',0,'DataSetOffset',0,'DataSetOffsetCheck',0,'DataSetLength',1,'DataSetLengthCheck',0,'EnableTriggerEvent',0,'TriggerMode',2,'TriggerLineOut',1,'ADCSWStartEnable',0,'SampleTime',-1,'SampleTimeCheck',1,'StatusPortEnable',0,'TLCFileName','rti120xadc_c1_adc')
  ADC_CLASS1_BL7 : rti1202lib_adc_class1/ADC_CLASS1_BL1  DSProperties=struct('RTI',struct('Version',uint32(1),'BlockType',struct('isSLSource',uint8(1),'isSLSink',uint8(1),'isHWSource',uint8(0),'isHWSink',uint8(1),'isSetup',uint8(0),'isInline',uint8(1),'isNonInline',uint8(0),'isInterrupt',uint8(0),'isChannelwise',uint8(1)),'IOBoardType',{{'DS120X','STD','ADCC1'}},'UnitType','ADC','Identifier','ADC','DialogType','ML','BlockSet','NONE','SlaveProcessor','NONE'))  RTIBlockInterface=struct('InputPortsActive',0,'InputPortsWidth',int32(1),'InputPortsDataType',{{'SS_BOOLEAN'}},'InputPortsName',{{'Continue'}},'OutputPortsActive',[1 1],'OutputPortsWidth',int32([1 1]),'OutputPortsDataType',{{'SS_DOUBLE','SS_INT16'}},'OutputPortsName',{{'ADC','Status'}},'DialogFcn','rti120xstdadcc1adcgui','SampleTime',{{-1}},'InitLevel',3,'IconTransparency','on','BlockDisplay',{{['ADC CL1\nChannel: 7'],'center'}},'BlockName',struct('Token',{{'ADC_CLASS1_BL1'}}))  RTIBlockParameters=struct('ReadMode',{{2,'OFF',[1 2]}},'ChannelNo',{{7,'OFF',[]}},'ConversionMode',{{1,'OFF',[1 2]}},'TriggerSource',{{2,'OFF',[1 2]}},'TriggerLineIn',{{1,'OFF',[1 16]}},'SampleMode',{{1,'OFF',[1 2]}},'BurstTriggerSource',{{1,'OFF',[1 2]}},'BurstTriggerLine',{{1,'OFF',[1 16]}},'ConvTriggerSource',{{3,'OFF',[1 3]}},'ConvTriggerLine',{{1,'OFF',[1 16]}},'ConvPeriod',{{'100e-6','OFF',[1e-6 1.34]}},'ConvPeriodCheck',{{0,'OFF',[]}},'BurstSize',{{'10','OFF',[]}},'BurstSizeCheck',{{0,'OFF',[]}},'DataSetOffset',{{'0','OFF',[]}},'DataSetOffsetCheck',{{0,'OFF',[]}},'DataSetLength',{{'1','OFF',[]}},'DataSetLengthCheck',{{0,'OFF',[]}},'EnableTriggerEvent',{{0,'OFF',[0 1]}},'TriggerMode',{{2,'OFF',[1 3]}},'TriggerLineOut',{{1,'OFF',[1 16]}},'ADCSWStartEnable',{{0,'OFF',[0 1]}},'SampleTime',{{'-1','OFF',[-1 inf]}},'SampleTimeCheck',{{0,'OFF',[]}},'StatusPortEnable',{{1,'OFF',[0 1]}},'TLCFileName',{{'rti120xadc_c1_adc','OFF',[]}})  RTISFcnParameters=struct('ReadMode','int16','ChannelNo','int16','ConversionMode','int16','TriggerSource','int16','TriggerLineIn','int16','SampleMode','int16','BurstTriggerSource','int16','BurstTriggerLine','int16','ConvTriggerSource','int16','ConvTriggerLine','int16','ConvPeriod','double','BurstSize','int16','DataSetOffset','int16','DataSetLength','int16','EnableTriggerEvent','int16','TriggerMode','int16','TriggerLineOut','int16','ADCSWStartEnable','int16','SampleTime','double','StatusPortEnable','int16','TLCFileName','char')  RTIBlockParaDefault=struct('ReadMode',1,'ChannelNo',1,'ConversionMode',1,'TriggerSource',1,'TriggerLineIn',1,'SampleMode',1,'BurstTriggerSource',1,'BurstTriggerLine',1,'ConvTriggerSource',3,'ConvTriggerLine',1,'ConvPeriod',0.0001,'ConvPeriodCheck',0,'BurstSize',10,'BurstSizeCheck',0,'DataSetOffset',0,'DataSetOffsetCheck',0,'DataSetLength',1,'DataSetLengthCheck',0,'EnableTriggerEvent',0,'TriggerMode',2,'TriggerLineOut',1,'ADCSWStartEnable',0,'SampleTime',-1,'SampleTimeCheck',1,'StatusPortEnable',0,'TLCFileName','rti120xadc_c1_adc')
  ADC_CLASS1_BL8 : rti1202lib_adc_class1/ADC_CLASS1_BL1  DSProperties=struct('RTI',struct('Version',uint32(1),'BlockType',struct('isSLSource',uint8(1),'isSLSink',uint8(1),'isHWSource',uint8(0),'isHWSink',uint8(1),'isSetup',uint8(0),'isInline',uint8(1),'isNonInline',uint8(0),'isInterrupt',uint8(0),'isChannelwise',uint8(1)),'IOBoardType',{{'DS120X','STD','ADCC1'}},'UnitType','ADC','Identifier','ADC','DialogType','ML','BlockSet','NONE','SlaveProcessor','NONE'))  RTIBlockInterface=struct('InputPortsActive',0,'InputPortsWidth',int32(1),'InputPortsDataType',{{'SS_BOOLEAN'}},'InputPortsName',{{'Continue'}},'OutputPortsActive',[1 1],'OutputPortsWidth',int32([1 1]),'OutputPortsDataType',{{'SS_DOUBLE','SS_INT16'}},'OutputPortsName',{{'ADC','Status'}},'DialogFcn','rti120xstdadcc1adcgui','SampleTime',{{-1}},'InitLevel',3,'IconTransparency','on','BlockDisplay',{{['ADC CL1\nChannel: 8'],'center'}},'BlockName',struct('Token',{{'ADC_CLASS1_BL1'}}))  RTIBlockParameters=struct('ReadMode',{{2,'OFF',[1 2]}},'ChannelNo',{{8,'OFF',[]}},'ConversionMode',{{1,'OFF',[1 2]}},'TriggerSource',{{2,'OFF',[1 2]}},'TriggerLineIn',{{1,'OFF',[1 16]}},'SampleMode',{{1,'OFF',[1 2]}},'BurstTriggerSource',{{1,'OFF',[1 2]}},'BurstTriggerLine',{{1,'OFF',[1 16]}},'ConvTriggerSource',{{3,'OFF',[1 3]}},'ConvTriggerLine',{{1,'OFF',[1 16]}},'ConvPeriod',{{'100e-6','OFF',[1e-6 1.34]}},'ConvPeriodCheck',{{0,'OFF',[]}},'BurstSize',{{'10','OFF',[]}},'BurstSizeCheck',{{0,'OFF',[]}},'DataSetOffset',{{'0','OFF',[]}},'DataSetOffsetCheck',{{0,'OFF',[]}},'DataSetLength',{{'1','OFF',[]}},'DataSetLengthCheck',{{0,'OFF',[]}},'EnableTriggerEvent',{{0,'OFF',[0 1]}},'TriggerMode',{{2,'OFF',[1 3]}},'TriggerLineOut',{{1,'OFF',[1 16]}},'ADCSWStartEnable',{{0,'OFF',[0 1]}},'SampleTime',{{'-1','OFF',[-1 inf]}},'SampleTimeCheck',{{0,'OFF',[]}},'StatusPortEnable',{{1,'OFF',[0 1]}},'TLCFileName',{{'rti120xadc_c1_adc','OFF',[]}})  RTISFcnParameters=struct('ReadMode','int16','ChannelNo','int16','ConversionMode','int16','TriggerSource','int16','TriggerLineIn','int16','SampleMode','int16','BurstTriggerSource','int16','BurstTriggerLine','int16','ConvTriggerSource','int16','ConvTriggerLine','int16','ConvPeriod','double','BurstSize','int16','DataSetOffset','int16','DataSetLength','int16','EnableTriggerEvent','int16','TriggerMode','int16','TriggerLineOut','int16','ADCSWStartEnable','int16','SampleTime','double','StatusPortEnable','int16','TLCFileName','char')  RTIBlockParaDefault=struct('ReadMode',1,'ChannelNo',1,'ConversionMode',1,'TriggerSource',1,'TriggerLineIn',1,'SampleMode',1,'BurstTriggerSource',1,'BurstTriggerLine',1,'ConvTriggerSource',3,'ConvTriggerLine',1,'ConvPeriod',0.0001,'ConvPeriodCheck',0,'BurstSize',10,'BurstSizeCheck',0,'DataSetOffset',0,'DataSetOffsetCheck',0,'DataSetLength',1,'DataSetLengthCheck',0,'EnableTriggerEvent',0,'TriggerMode',2,'TriggerLineOut',1,'ADCSWStartEnable',0,'SampleTime',-1,'SampleTimeCheck',1,'StatusPortEnable',0,'TLCFileName','rti120xadc_c1_adc')
  Bus Creator4 : BusCreator  Inputs=3
  Bus Creator6 : BusCreator  Inputs=12
  Gain{,1..7,12,22..29} (17 alike) : Gain
  Gain{8..11} (4 alike) : Gain  Gain=6
  Gain{13..18,20..21} (8 alike) : Gain  Gain=10
  Ground{,1..7} (8 alike) : Ground
  Sum10 : Sum  Inputs=|+-
  Sum11 : Sum  Inputs=|+-
  Sum9 : Sum  Inputs=|+-
  Terminator{,1..16} (17 alike) : Terminator
  i_c_offset : Constant  Value=-0.13
  "volt->amp_i_a           " : Gain  Gain=-12
  volt->amp_i_b : Gain  Gain=-12
  volt->amp_i_c : Gain  Gain=-12
  i(a,b,c)[A] : Outport  VectorParamsAs1DForOutWhenUnconnected=off
  AD_values[V] : Outport  Port=2  VectorParamsAs1DForOutWhenUnconnected=off
  wires:
  Gain18/1 -> Bus Creator6/10, volt->amp_i_c/1  "Voltage ADC7[V]"
  Gain17/1 -> Bus Creator6/7, volt->amp_i_b/1  "Voltage ADC5[V]"
  Gain13/1 -> Bus Creator6/1, "volt->amp_i_a           "/1  "Voltage ADC1[V]"
  "volt->amp_i_a           "/1 -> Sum9/1
  volt->amp_i_b/1 -> Sum10/1
  volt->amp_i_c/1 -> Sum11/1
  Sum11/1 -> Bus Creator4/3  "current Phase C [A]"
  Sum10/1 -> Bus Creator4/2  "current Phase B [A]"
  Sum9/1 -> Bus Creator4/1  "current Phase A [A]"
  i_c_offset/1 -> Sum11/2
  " i_a_offset"/1 -> Sum9/2
  " i_b_offset  "/1 -> Sum10/2
  Gain21/1 -> Gain11/1, Bus Creator6/11  "Voltage ADC8[V]"
  Bus Creator4/1 -> i(a,b,c)[A]/1
  Gain15/1 -> Bus Creator6/4, Gain9/1  "Voltage ADC3[V]"
  Gain14/1 -> Bus Creator6/2, Gain8/1  "Voltage ADC2[V]"
  Gain16/1 -> Gain12/1, Bus Creator6/6  "Voltage ADC4[V]"
  Gain20/1 -> Gain10/1, Bus Creator6/8  "Voltage ADC6[V]"
  Bus Creator6/1 -> AD_values[V]/1
  Gain/1 -> Terminator/1
  Ground/1 -> Gain/1  "Overflow_ADC1"
  Ground1/1 -> Gain1/1  "Overflow_ADC5"
  Gain1/1 -> Terminator1/1
  Ground2/1 -> Gain2/1  "Overflow_ADC7"
  Gain2/1 -> Terminator2/1
  Ground3/1 -> Gain3/1  "Overflow_ADC2"
  Gain3/1 -> Terminator3/1
  Ground4/1 -> Gain4/1  "Overflow_ADC3"
  Gain4/1 -> Terminator4/1
  Ground5/1 -> Gain5/1  "Overflow_ADC4"
  Gain5/1 -> Terminator5/1
  Ground6/1 -> Gain6/1  "Overflow_ADC6"
  Gain6/1 -> Terminator6/1
  Ground7/1 -> Gain7/1  "Overflow_ADC8"
  Gain7/1 -> Terminator7/1
  Gain8/1 -> Bus Creator6/3  "PhaseA_Voltage[V]"
  Gain10/1 -> Bus Creator6/9  "PhaseB_Voltage[V]"
  Gain11/1 -> Bus Creator6/12  "PhaseC_Voltage[V]"
  Gain9/1 -> Bus Creator6/5  "Battery_Voltage[V]"
  Gain12/1 -> Terminator12/1  "not_used"
  ADC_CLASS1_BL1/1 -> Gain13/1
  ADC_CLASS1_BL2/1 -> Gain14/1
  ADC_CLASS1_BL3/1 -> Gain15/1
  ADC_CLASS1_BL4/1 -> Gain16/1
  ADC_CLASS1_BL5/1 -> Gain17/1
  ADC_CLASS1_BL7/1 -> Gain18/1
  ADC_CLASS1_BL6/1 -> Gain20/1
  ADC_CLASS1_BL8/1 -> Gain21/1
  Gain22/1 -> Terminator8/1
  Gain23/1 -> Terminator9/1
  Gain24/1 -> Terminator10/1
  Gain25/1 -> Terminator11/1
  Gain26/1 -> Terminator13/1
  Gain27/1 -> Terminator14/1
  Gain28/1 -> Terminator15/1
  Gain29/1 -> Terminator16/1
  ADC_CLASS1_BL8/2 -> Gain29/1
  ADC_CLASS1_BL6/2 -> Gain28/1
  ADC_CLASS1_BL4/2 -> Gain27/1
  ADC_CLASS1_BL3/2 -> Gain26/1
  ADC_CLASS1_BL2/2 -> Gain25/1
  ADC_CLASS1_BL7/2 -> Gain24/1
  ADC_CLASS1_BL5/2 -> Gain23/1  "ADC_CL1_CH5_Status"
  ADC_CLASS1_BL1/2 -> Gain22/1  "ADC_CL1_CH1_Status"

== system BLDC_Demo/Control/Input/DISCRETE_PT1 ==
  Reset[0|1] : Inport
  In : Inport  Port=2
  K : Inport  Port=3
  T[s] : Inport  Port=4
  T_Sample[s] : Inport  Port=5
  1|FilterTime : Product  Inputs=*/  SaturateOnIntegerOverflow=on  InputSameDT=on  OutDataTypeStr=Inherit: Same as first input
  Proportional : Product  Inputs=**  SaturateOnIntegerOverflow=on  InputSameDT=on  OutDataTypeStr=Inherit: Same as first input
  Sum : Sum  Inputs=-+|  SaturateOnIntegerOverflow=on  InputSameDT=on  OutDataTypeStr=Inherit: Same as first input
  Unit Delay : UnitDelay  SampleTime=-1  HasFrameUpgradeWarning=on
  discrete_Integrator_Init : Subsystem  mask(DISCRETE_INTEGRATOR){upper_limit=upper_limit_int, lower_limit=lower_limit_int, ASMProperties=struct('Name','discrete_integrator','Version','1.0','Library','ASM_ElectricComponents_lib')}
      mask prompts: upper_limit "upper limit"; lower_limit "lower limit"
      mask help: (c) Copyright 2007, dSPACE GmbH. All rights reserved.
      mask Help: eval(['asm_modelhelp(gcbh)'])
  zero : Constant  Value=0  SampleTime=-1
  Out : Outport  VectorParamsAs1DForOutWhenUnconnected=off
  wires:
  In/1 -> Proportional/1
  Sum/1 -> discrete_Integrator_Init/2(In)
  K/1 -> Proportional/2
  Proportional/1 -> Sum/2
  discrete_Integrator_Init/1(Out) -> 1|FilterTime/1
  1|FilterTime/1 -> Out/1, Unit Delay/1
  Unit Delay/1 -> Sum/1
  T[s]/1 -> 1|FilterTime/2
  Reset[0|1]/1 -> discrete_Integrator_Init/1(Reset[0|1])
  T_Sample[s]/1 -> discrete_Integrator_Init/4(T_Sample[s])
  zero/1 -> discrete_Integrator_Init/3(Initial)

== system BLDC_Demo/Control/Input/Rename and Convert ==
  In1 : Inport
  In2 : Inport  Port=2
  In3 : Inport  Port=3
  In4 : Inport  Port=4
  In5 : Inport  Port=5
  In6 : Inport  Port=6
  bool2double{1..6} (6 alike) : DataTypeConversion
  Out1 : Outport  VectorParamsAs1DForOutWhenUnconnected=off
  Out2 : Outport  Port=2  VectorParamsAs1DForOutWhenUnconnected=off
  Out3 : Outport  Port=3  VectorParamsAs1DForOutWhenUnconnected=off
  Out4 : Outport  Port=4  VectorParamsAs1DForOutWhenUnconnected=off
  Out5 : Outport  Port=5  VectorParamsAs1DForOutWhenUnconnected=off
  Out6 : Outport  Port=6  VectorParamsAs1DForOutWhenUnconnected=off
  wires:
  In1/1 -> bool2double1/1
  In2/1 -> bool2double2/1
  In3/1 -> bool2double3/1
  In4/1 -> bool2double4/1
  In5/1 -> bool2double5/1
  In6/1 -> bool2double6/1
  bool2double1/1 -> Out1/1
  bool2double2/1 -> Out2/1
  bool2double3/1 -> Out3/1
  bool2double4/1 -> Out4/1
  bool2double5/1 -> Out5/1
  bool2double6/1 -> Out6/1

== system BLDC_Demo/Control/Input/SignalCollector ==
  BusCreator : BusCreator  Inputs=1
  tag scope: BUS_Inputs=global
  wires:
  [BUS_PMSM_IN] -> BusCreator/1
  BusCreator/1 -> [BUS_Inputs]  "Inputs"

== system BLDC_Demo/Control/Input/dummy_hall_signals ==
  Ground1 : Ground
  hall_freqbased_vel : Outport  VectorParamsAs1DForOutWhenUnconnected=off
  wires:
  Ground1/1 -> hall_freqbased_vel/1  "hall_freqbased_vel"

== system BLDC_Demo/Control/Input/mech2elec ==
  elec. Angle Offset : Inport
  mech angle : Inport  Port=2
  Constant4 : Constant  Value=360
  Gain3 : Gain  Gain=4
  Math Function : Math  Operator=mod  SaturateOnIntegerOverflow=on
  Sum : Sum  Inputs=|++
  elec angle : Outport  VectorParamsAs1DForOutWhenUnconnected=off
  wires:
  elec. Angle Offset/1 -> Sum/1
  Gain3/1 -> Sum/2
  Sum/1 -> Math Function/1
  Math Function/1 -> elec angle/1  "Inc_elec_pos"
  Constant4/1 -> Math Function/2
  mech angle/1 -> Gain3/1
